simulink model "R19_Modelo_control_1GDL_Bancada"  (R2021b)
settings: Solver=ode45  StartTime=0.0  StopTime=7  RelTol=1e-3
values from neighbouring files (symbols this model uses):
  airgap = r.air_gap/1000    [CONTROL_1GDL_BANCADA.m]
  current_I = r.current(1,2:32)    [CONTROL_1GDL_BANCADA.m]
  dtCurrent = 1e-4    (= 0.0001)    [CONTROL_1GDL_BANCADA.m]
  dTSensor = 5e-4    (= 0.0005)    [CONTROL_1GDL_BANCADA.m]
  g = 9.81    [CONTROL_1GDL_BANCADA.m]
  Imax = 40    [CONTROL_1GDL_BANCADA.m]
  Imin = -40    [CONTROL_1GDL_BANCADA.m]
  inductance = r.inductance    [CONTROL_1GDL_BANCADA.m]
  K_d = place(Ad2,Bd2,polos_dis)    [CONTROL_1GDL_BANCADA.m]
  Ki = 100    [CONTROL_1GDL_BANCADA.m]
  Kp = 25    [CONTROL_1GDL_BANCADA.m]
  m = 122/6    (= 20.3333333333)    [CONTROL_1GDL_BANCADA.m]
  noiseSensor = 1.4819e-5    (= 1.4819e-05)    [CONTROL_1GDL_BANCADA.m]
  Rcoil = 0.319    [CONTROL_1GDL_BANCADA.m]
  T = 0.002    [CONTROL_1GDL_BANCADA.m]
  VarianceCurrentNoise = 0.4^2    (= 0.16)    [CONTROL_1GDL_BANCADA.m]
  Vmax = 48    [CONTROL_1GDL_BANCADA.m]
  Vmin = -48    [CONTROL_1GDL_BANCADA.m]
  z0 = 17.5*1e-3    (= 0.0175)    [CONTROL_1GDL_BANCADA.m]
undefined symbols (not defined in the file or in its folder): DiscIntNeverNeededParam, resCurrent
libraries: cstblocks x3, spsPWMGeneratorDCDCLib x2, slpidlib x1
settings Model: Creator=skapa  LastModifiedBy=emate
settings SolverCC: AlgebraicLoopSolver=TrustRegion
settings DataIOCC: LimitDataPoints=on  SaveFormat=Array  SignalLoggingSaveFormat=ModelDataLogs  ReturnWorkspaceOutputs=off
settings OptimizationCC: BlockReduction=off  BooleanDataType=off  LifeSpan=inf
settings DebuggingCC: SaveWithParameterizedLinksMsg=none  UnderspecifiedInitializationDetection=Classic  MergeDetectMultiDrivingBlocksExec=none  SignalResolutionControl=TryResolveAllWithWarning  MultiTaskDSMMsg=warning  MultiTaskCondExecSysMsg=none  SFUnexpectedBacktrackingDiag=warning  SFNoUnconditionalDefaultTransitionDiag=warning  SFExecutionAtInitializationDiag=none  SFMachineParentedDataDiag=warning  ArithmeticOperatorsInVariantConditions=warning
settings HardwareCC: ProdBitPerPointer=32  ProdBitPerSizeT=32  ProdBitPerPtrDiffT=32  ProdLargestAtomicFloat=None  ProdIntDivRoundTo=Undefined  ProdEndianess=Unspecified  ProdWordSize=32  ProdHWDeviceType=32-bit Generic  TargetUnknown=on
settings ModelReferenceCC: PropagateSignalLabelsOutOfModel=off
settings SFSimCC: SimUseLocalCustomCode=off  CustomCodeUndefinedFunction=UseInterfaceOnly
settings RTWCC: RTWUseLocalCustomCode=off
settings CodeAppCC: StateflowObjectComments=on
settings GRTTargetCC: TargetLangStandard=C89/C90 (ANSI)
settings ConfigComp: CovMetricSettings=dw  CovSaveCumulativeToWorkspaceVar=on  CovSaveSingleToWorkspaceVar=on  CovExternalEMLEnable=off

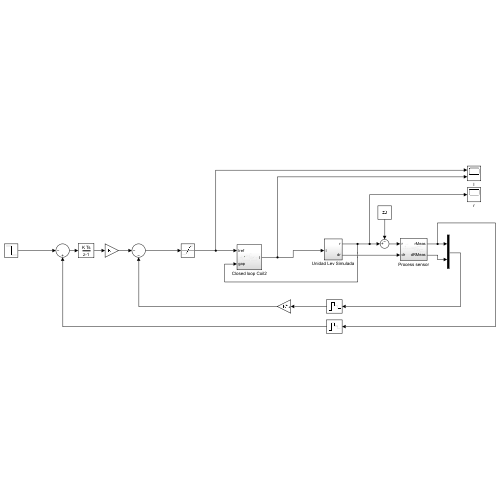
[thumbnail: Simulink's stored preview of the top-level diagram]
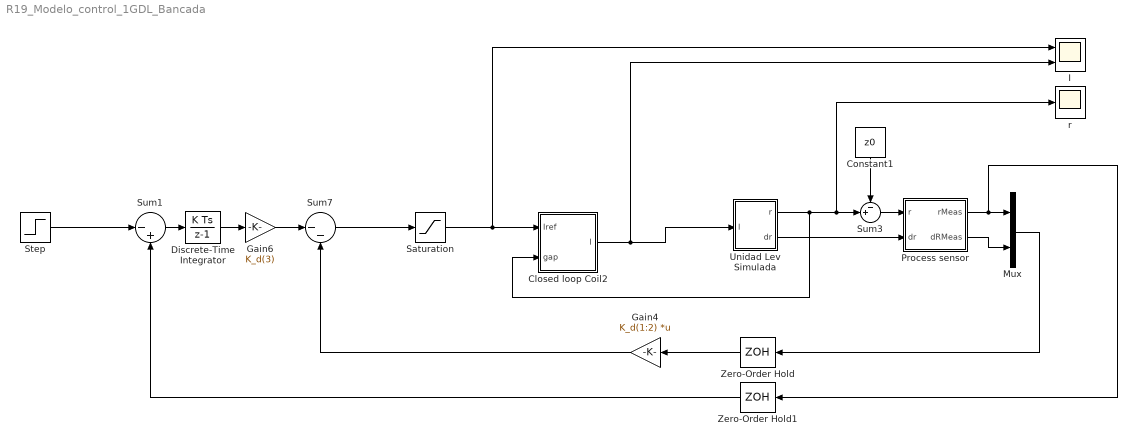
== system R19_Modelo_control_1GDL_Bancada ==
  Closed loop Coil2 : Subsystem
  Constant1 : Constant  Value=z0  SampleTime=T
  Discrete-Time Integrator : DiscreteIntegrator  SampleTime=T  ICPrevOutput=DiscIntNeverNeededParam  ICPrevScaledInput=DiscIntNeverNeededParam
  Gain4 : Gain  Gain=K_d(1:2)  Multiplication=Matrix(K*u)
  Gain6 : Gain  Gain=K_d(3)
  I : Scope  NumInputPorts=2
  Mux : Mux  Inputs=2
  Process sensor : Subsystem
  Saturation : Saturate  UpperLimit=Imax  LowerLimit=Imin
  Step : Step  After=-1e-3  SampleTime=T
  Sum1 : Sum  Inputs=|-+
  Sum3 : Sum  Inputs=-+|
  Sum7 : Sum  Inputs=|--
  Unidad Lev Simulada : Subsystem
  Zero-Order Hold : ZeroOrderHold  SampleTime=T
  Zero-Order Hold1 : ZeroOrderHold  SampleTime=T
  r : Scope
  wires:
  Sum1/1 -> Discrete-Time Integrator/1
  Unidad Lev Simulada/1(r) -> Closed loop Coil2/2(gap), Sum3/2, r/1
  Discrete-Time Integrator/1 -> Gain6/1
  Gain6/1 -> Sum7/1
  Gain4/1 -> Sum7/2
  Constant1/1 -> Sum3/1
  Zero-Order Hold/1 -> Gain4/1
  Sum7/1 -> Saturation/1
  Sum3/1 -> Process sensor/1(r)
  Mux/1 -> Zero-Order Hold/1
  Zero-Order Hold1/1 -> Sum1/2
  Unidad Lev Simulada/2(dr) -> Process sensor/2(dr)
  Process sensor/1(rMeas) -> Zero-Order Hold1/1, Mux/1
  Process sensor/2(dRMeas) -> Mux/2
  Step/1 -> Sum1/1
  Saturation/1 -> Closed loop Coil2/1(Iref), I/1
  Closed loop Coil2/1(I) -> I/2, Unidad Lev Simulada/1(I)

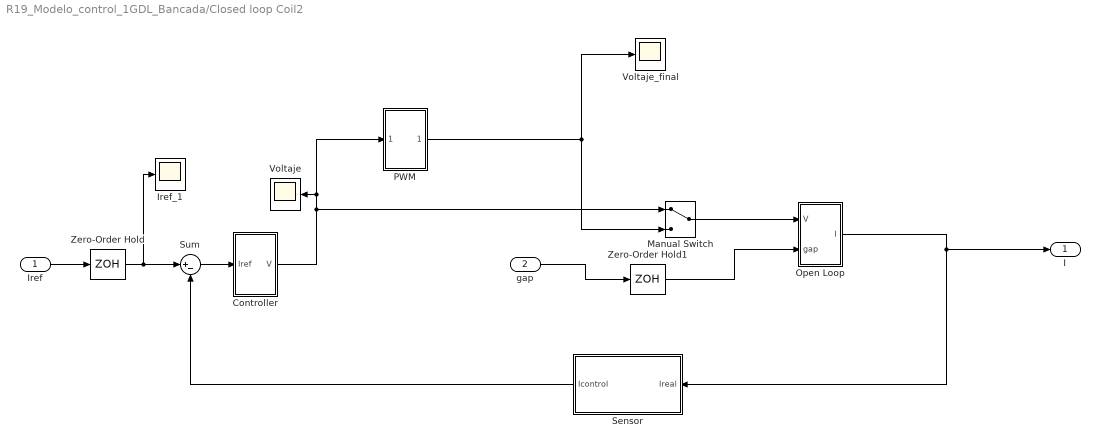
== system R19_Modelo_control_1GDL_Bancada/Closed loop Coil2 ==
  Iref : Inport
  gap : Inport  Port=2
  Controller : Subsystem
  Iref_1 : Scope
  Manual Switch : ManualSwitch
  Open Loop : Subsystem
  PWM : Subsystem
  Sensor : Subsystem
  Sum : Sum  Inputs=|+-
  Voltaje : Scope
  Voltaje_final : Scope
  Zero-Order Hold : ZeroOrderHold  SampleTime=dtCurrent
  Zero-Order Hold1 : ZeroOrderHold  SampleTime=dtCurrent
  I : Outport
  wires:
  Controller/1(V) -> Manual Switch/1, PWM/1(In2), Voltaje/1
  Open Loop/1(I) -> Sensor/1(Ireal), I/1
  Iref/1 -> Zero-Order Hold/1
  Sum/1 -> Controller/1(Iref)
  Sensor/1(Icontrol) -> Sum/2
  gap/1 -> Zero-Order Hold1/1
  Zero-Order Hold/1 -> Iref_1/1, Sum/1
  Zero-Order Hold1/1 -> Open Loop/2(gap)
  Manual Switch/1 -> Open Loop/1(V)
  PWM/1(Out1) -> Voltaje_final/1, Manual Switch/2

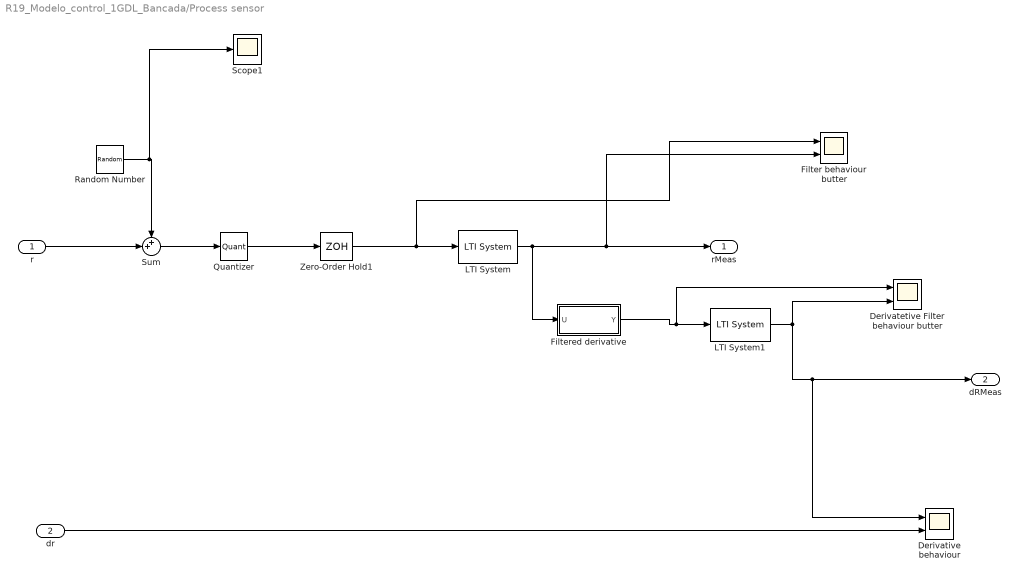
== system R19_Modelo_control_1GDL_Bancada/Process sensor ==
  r : Inport
  dr : Inport  Port=2
  Derivatetive Filter behaviour butter : Scope  NumInputPorts=2
  Derivative behaviour : Scope  NumInputPorts=2
  Filter behaviour butter : Scope  NumInputPorts=2
  Filtered derivative : Subsystem
  LTI System : cstblocks/LTI System  sys=Airgap_filter  IC=[]
  LTI System1 : cstblocks/LTI System  sys=Derivative_filter  IC=[]
  Quantizer : Quantizer  QuantizationInterval=resSensor
  Random Number : RandomNumber  Variance=noiseSensor^2
  Scope1 : Scope
  Sum : Sum  Inputs=++|
  Zero-Order Hold1 : ZeroOrderHold  SampleTime=dTSensor
  rMeas : Outport
  dRMeas : Outport  Port=2
  wires:
  r/1 -> Sum/2
  Random Number/1 -> Sum/1, Scope1/1
  Sum/1 -> Quantizer/1
  Quantizer/1 -> Zero-Order Hold1/1
  Zero-Order Hold1/1 -> Filter behaviour butter/1, LTI System/1
  Filtered derivative/1(Y) -> LTI System1/1, Derivatetive Filter behaviour butter/1
  dr/1 -> Derivative behaviour/2
  LTI System/1 -> rMeas/1, Filter behaviour butter/2, Filtered derivative/1(U)
  LTI System1/1 -> Derivative behaviour/1, dRMeas/1, Derivatetive Filter behaviour butter/2

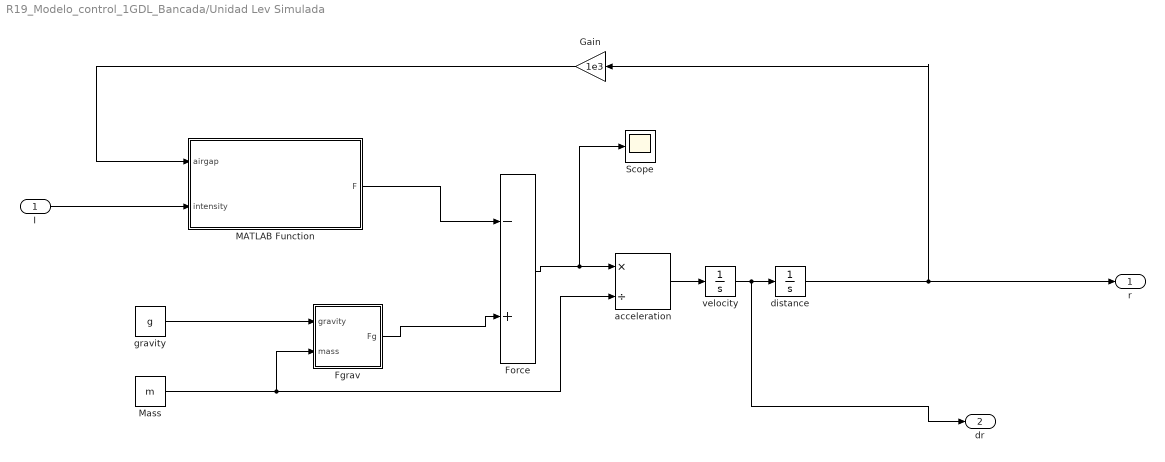
== system R19_Modelo_control_1GDL_Bancada/Unidad Lev Simulada ==
  I : Inport
  Fgrav : Subsystem
  Force : Sum  Inputs=-+
  Gain : Gain  Gain=1e3
  MATLAB Function : MATLAB Function  TreatAsAtomicUnit=on
  Mass : Constant  Value=m
  Scope : Scope
  acceleration : Product  Inputs=*/
  distance : Integrator  InitialCondition=z0
  gravity : Constant  Value=g
  velocity : Integrator
  r : Outport  VectorParamsAs1DForOutWhenUnconnected=off
  dr : Outport  Port=2  VectorParamsAs1DForOutWhenUnconnected=off
  wires:
  Force/1 -> Scope/1, acceleration/1
  MATLAB Function/1(F) -> Force/1
  Fgrav/1(Fg) -> Force/2
  gravity/1 -> Fgrav/1(gravity)
  acceleration/1 -> velocity/1
  Mass/1 -> Fgrav/2(mass), acceleration/2
  I/1 -> MATLAB Function/2(intensity)
  velocity/1 -> dr/1, distance/1
  distance/1 -> Gain/1, r/1
  Gain/1 -> MATLAB Function/1(airgap)

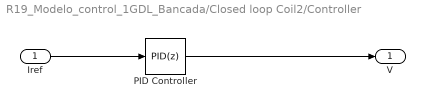
== system R19_Modelo_control_1GDL_Bancada/Closed loop Coil2/Controller ==
  Iref : Inport
  PID Controller : slpidlib/PID Controller  Controller=PID  Form=Parallel  TimeDomain=Discrete-time  UseExternalTs=off  SampleTime=dtCurrent  IntegratorMethod=Forward Euler  FilterMethod=Forward Euler  ControllerParametersSource=internal  P=Kp  I=Ki  D=0  UseFilter=on  N=100  TunerSelectOption=Transfer Function Based (PID Tuner App)  InitialConditionSource=internal  InitialConditionForIntegrator=0  InitialConditionForFilter=0  DifferentiatorICPrevScaledInput=0  ExternalReset=none  TrackingMode=off  Kt=1  LimitOutput=on  SatLimitsSource=internal  UpperSaturationLimit=Vmax  LowerSaturationLimit=Vmin  LinearizeAsGain=on  AntiWindupMode=clamping  Kb=1  POutMin=[]  POutMax=[]  IOutMin=[]  IOutMax=[]  DOutMin=[]  DOutMax=[]  NOutMin=[]  NOutMax=[]  SumOutMin=[]  SumOutMax=[]  SaturationOutMin=[]  SaturationOutMax=[]  PParamMin=[]  PParamMax=[]  IParamMin=[]  IParamMax=[]  DParamMin=[]  DParamMax=[]  NParamMin=[]  NParamMax=[]  KbParamMin=[]  KbParamMax=[]  KtParamMin=[]  KtParamMax=[]  KbOutMin=[]  KbOutMax=[]  KtOutMin=[]  KtOutMax=[]  IntegratorOutMin=[]  IntegratorOutMax=[]  FilterOutMin=[]  FilterOutMax=[]  SumI1OutMin=[]  SumI1OutMax=[]  SumI2OutMin=[]  SumI2OutMax=[]  SumI3OutMin=[]  SumI3OutMax=[]  SumI4OutMin=[]  SumI4OutMax=[]  SumDOutMin=[]  SumDOutMax=[]  DifferentiatorOutMin=[]  DifferentiatorOutMax=[]  FilterDiffOutCoefMin=[]  FilterDiffOutCoefMax=[]  ReciprocalOutMin=[]  ReciprocalOutMax=[]  SumDenOutMin=[]  SumDenOutMax=[]  SumNumOutMin=[]  SumNumOutMax=[]  DivideOutMin=[]  DivideOutMax=[]  UdiffTsProdOutMin=[]  UdiffTsProdOutMax=[]  NTsProdOutMin=[]  NTsProdOutMax=[]  UintegralTsProdOutMin=[]  UintegralTsProdOutMax=[]  UngainTsProdOutMin=[]  UngainTsProdOutMax=[]  IntegratorContinuousStateAttributes=''  IntegratorStateMustResolveToSignalObject=off  IntegratorRTWStateStorageClass=Auto  FilterContinuousStateAttributes=''  FilterStateMustResolveToSignalObject=off  FilterRTWStateStorageClass=Auto  ParallelPVariant=InternalParameters  IdealPVariant=Disabled  IVariant=InternalParameters  DVariant=InternalParameters  IntegratorVariant=Discrete  SatVariant=Enabled  AWVariant=DiscClampingParallel  PCopyVariant=Disabled  TRVariant=Disabled  FdbkBlocksVariant=Forward  IdealPFdbkVariant=Disabled  SatFdbkVariant=Disabled  DerivativeFilterVariant=ForwardEulerFilter  NVariant=InternalParameters  NCopyVariant=Disabled  FilterICVariant=InternalICsFilter  IntegratorICVariant=InternalICs  ExternalResetVariant=Disabled  TRSumVariant=Passthrough  SumFdbkVariant=Disabled  SumVariant=Sum_PID  TsampFilterVariant=InternalTs  TsampNgainVariant=Passthrough  TsampIntegralVariant=Passthrough  ExternalSaturationOutDataTypeStr=Inherit: Same as second input
  V : Outport
  wires:
  Iref/1 -> PID Controller/1
  PID Controller/1 -> V/1

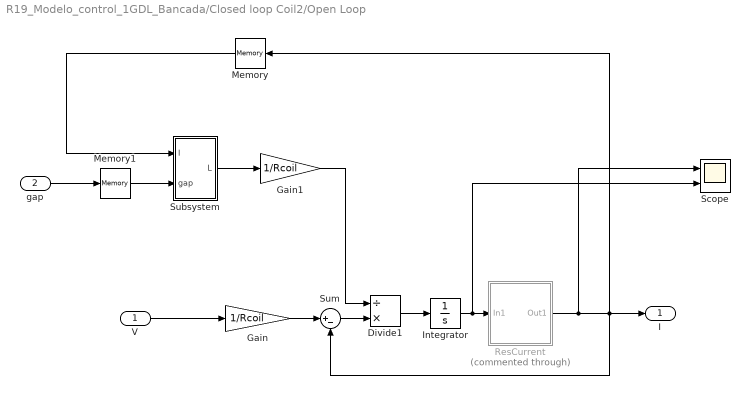
== system R19_Modelo_control_1GDL_Bancada/Closed loop Coil2/Open Loop ==
  V : Inport
  gap : Inport  Port=2
  Divide1 : Product  Inputs=/*
  Gain : Gain  Gain=1/Rcoil
  Gain1 : Gain  Gain=1/Rcoil
  Integrator : Integrator
  Memory : Memory
  Memory1 : Memory
  ResCurrent : Subsystem  Commented=through
  Scope : Scope  NumInputPorts=2
  Subsystem : Subsystem
  Sum : Sum  Inputs=|+-
  I : Outport
  wires:
  V/1 -> Gain/1
  Gain1/1 -> Divide1/1
  Gain/1 -> Sum/1
  Sum/1 -> Divide1/2
  Divide1/1 -> Integrator/1
  Subsystem/1(L) -> Gain1/1
  Memory/1 -> Subsystem/1(I)
  gap/1 -> Memory1/1
  ResCurrent/1(Out1) -> Scope/1, Sum/2, Memory/1, I/1
  Integrator/1 -> Scope/2, ResCurrent/1(In1)
  Memory1/1 -> Subsystem/2(gap)

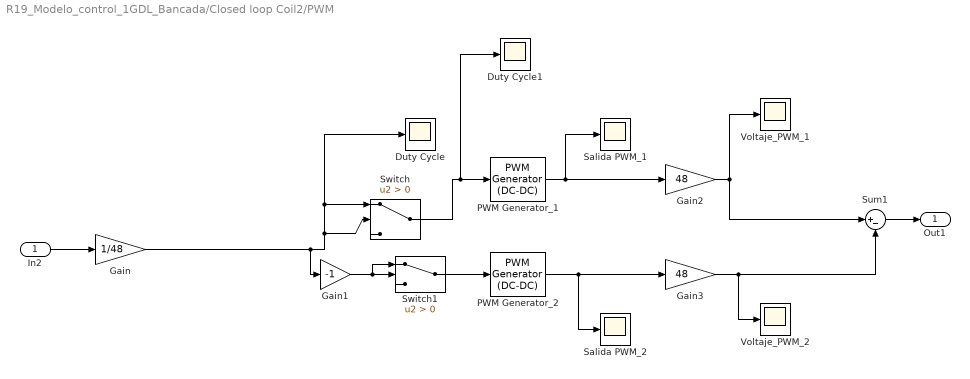
== system R19_Modelo_control_1GDL_Bancada/Closed loop Coil2/PWM ==
  In2 : Inport
  Duty Cycle : Scope
  Duty Cycle1 : Scope
  Gain : Gain  Gain=1/48
  Gain1 : Gain  Gain=-1
  Gain2 : Gain  Gain=48
  Gain3 : Gain  Gain=48
  PWM Generator_1 : spsPWMGeneratorDCDCLib/PWM Generator (DC-DC)  Fsw=20000  Ts=1/20000
  PWM Generator_2 : spsPWMGeneratorDCDCLib/PWM Generator (DC-DC)  Fsw=20000  Ts=1/20000
  Salida PWM_1 : Scope
  Salida PWM_2 : Scope
  Sum1 : Sum  Inputs=|+-
  Switch : Switch  Criteria=u2 > Threshold
  Switch1 : Switch  Criteria=u2 > Threshold
  Voltaje_PWM_1 : Scope
  Voltaje_PWM_2 : Scope
  Out1 : Outport
  wires:
  Gain2/1 -> Sum1/1, Voltaje_PWM_1/1
  PWM Generator_1/1 -> Gain2/1, Salida PWM_1/1
  Gain/1 -> Gain1/1, Switch/1, Duty Cycle/1, Switch/2
  Sum1/1 -> Out1/1
  PWM Generator_2/1 -> Gain3/1, Salida PWM_2/1
  Gain1/1 -> Switch1/2, Switch1/1
  Switch1/1 -> PWM Generator_2/1
  Gain3/1 -> Sum1/2, Voltaje_PWM_2/1
  Switch/1 -> PWM Generator_1/1, Duty Cycle1/1
  In2/1 -> Gain/1

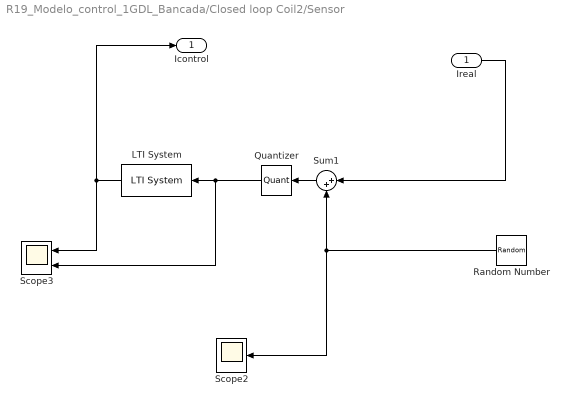
== system R19_Modelo_control_1GDL_Bancada/Closed loop Coil2/Sensor ==
  Ireal : Inport
  LTI System : cstblocks/LTI System  sys=Current_filter  IC=[]
  Quantizer : Quantizer  QuantizationInterval=resCurrentSensor
  Random Number : RandomNumber  Variance=VarianceCurrentNoise
  Scope2 : Scope
  Scope3 : Scope  NumInputPorts=2
  Sum1 : Sum  Inputs=|++
  Icontrol : Outport
  wires:
  Random Number/1 -> Scope2/1, Sum1/2
  Ireal/1 -> Sum1/1
  Sum1/1 -> Quantizer/1
  Quantizer/1 -> Scope3/2, LTI System/1
  LTI System/1 -> Scope3/1, Icontrol/1

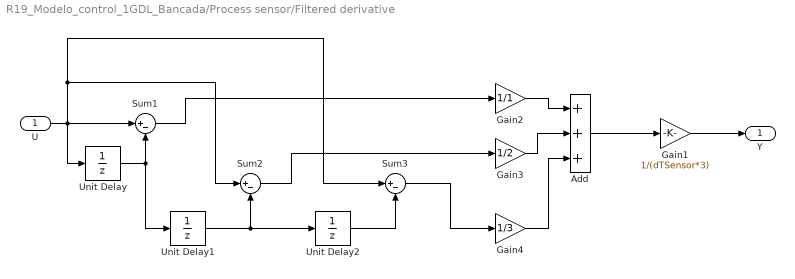
== system R19_Modelo_control_1GDL_Bancada/Process sensor/Filtered derivative ==
  U : Inport
  Add : Sum  Inputs=+++
  Gain1 : Gain  Gain=1/(dTSensor*3)
  Gain2 : Gain  Gain=1/1
  Gain3 : Gain  Gain=1/2
  Gain4 : Gain  Gain=1/3
  Sum1 : Sum  Inputs=|+-
  Sum2 : Sum  Inputs=|+-
  Sum3 : Sum  Inputs=|+-
  Unit Delay : UnitDelay  SampleTime=-1  HasFrameUpgradeWarning=on
  Unit Delay1 : UnitDelay  SampleTime=-1  HasFrameUpgradeWarning=on
  Unit Delay2 : UnitDelay  SampleTime=-1  HasFrameUpgradeWarning=on
  Y : Outport
  wires:
  U/1 -> Sum1/1, Sum2/1, Sum3/1, Unit Delay/1
  Unit Delay/1 -> Sum1/2, Unit Delay1/1
  Unit Delay2/1 -> Sum3/2
  Unit Delay1/1 -> Unit Delay2/1, Sum2/2
  Add/1 -> Gain1/1
  Gain1/1 -> Y/1
  Gain4/1 -> Add/3
  Gain3/1 -> Add/2
  Gain2/1 -> Add/1
  Sum1/1 -> Gain2/1
  Sum2/1 -> Gain3/1
  Sum3/1 -> Gain4/1

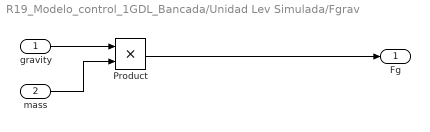
== system R19_Modelo_control_1GDL_Bancada/Unidad Lev Simulada/Fgrav ==
  gravity : Inport
  mass : Inport  Port=2
  Product : Product
  Fg : Outport  VectorParamsAs1DForOutWhenUnconnected=off
  wires:
  Product/1 -> Fg/1
  gravity/1 -> Product/1
  mass/1 -> Product/2

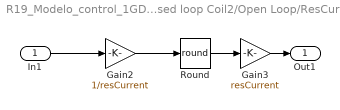
== system R19_Modelo_control_1GDL_Bancada/Closed loop Coil2/Open Loop/ResCurrent ==
  In1 : Inport
  Gain2 : Gain  Gain=1/resCurrent
  Gain3 : Gain  Gain=resCurrent
  Round : Rounding  Operator=round
  Out1 : Outport
  wires:
  Round/1 -> Gain3/1
  Gain3/1 -> Out1/1
  Gain2/1 -> Round/1
  In1/1 -> Gain2/1

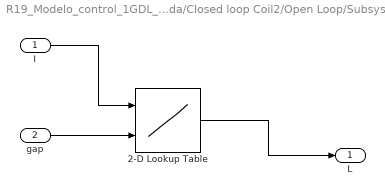
== system R19_Modelo_control_1GDL_Bancada/Closed loop Coil2/Open Loop/Subsystem ==
  I : Inport
  gap : Inport  Port=2
  2-D Lookup Table : Lookup_n-D  BreakpointsForDimension1=current_I  BreakpointsForDimension2=airgap  Table=inductance  InternalRulePriority=Speed  RndMeth=Simplest  InputSameDT=on
      settings: InputPortMap=u0,u1
  L : Outport
  wires:
  2-D Lookup Table/1 -> L/1
  I/1 -> 2-D Lookup Table/1
  gap/1 -> 2-D Lookup Table/2

== matlab function R19_Modelo_control_1GDL_Bancada/Unidad Lev Simulada/MATLAB Function ==
  data: airgap input; F output; intensity input
function F = HEMSlev1DOF(airgap, intensity)
% Computes the levitation force (N) of all the HEMS units as a function of 
% their air gaps (mm) and intensities (A)
% ═════════════════════════════════════════════════════════════════════════
% Last updated: 01.15.2021
% ════════════════════════════════════════════════════════════════════════

x   = airgap;
y   = intensity;

p00 =       926.8;
p10 =       -62.3;
p01 =       10.82;
p20 =       1.203;
p11 =     -0.4806;
p02 =    -0.06986;
p21 =    0.007783;
p12 =    0.002722;
p03 =   -0.001275;

F = p00 + ...
    p10*x + ...
    p01*y + ...
    p20*x^2 + ...
    p11*x*y + ...
    p02*y^2 + ...
    p21*x^2*y + ...
    p12*x*y^2 + ...
    p03*y^3;
